simulink library "PB_Library_Master"  (R2020b)
settings: Solver=VariableStepAuto  StartTime=0.0  StopTime=10.0  RelTol=1e-3
undefined symbols (not defined in the file): A_M, B_M, E0_M, f_sw, K_M, Q_M, Q_rr, r_c, r_D, R_M, SOC_Init_M, u_ce0, u_D0
libraries: $bdroot x7, Lib_PF_BusLoadDC_TMATS x3, Lib_Dyn_StateSpace_EMTAT x3, TemperatureBlock x1
(part 1 of 3)
settings Model: Creator=nbutler2  LastModifiedBy=nbutler2

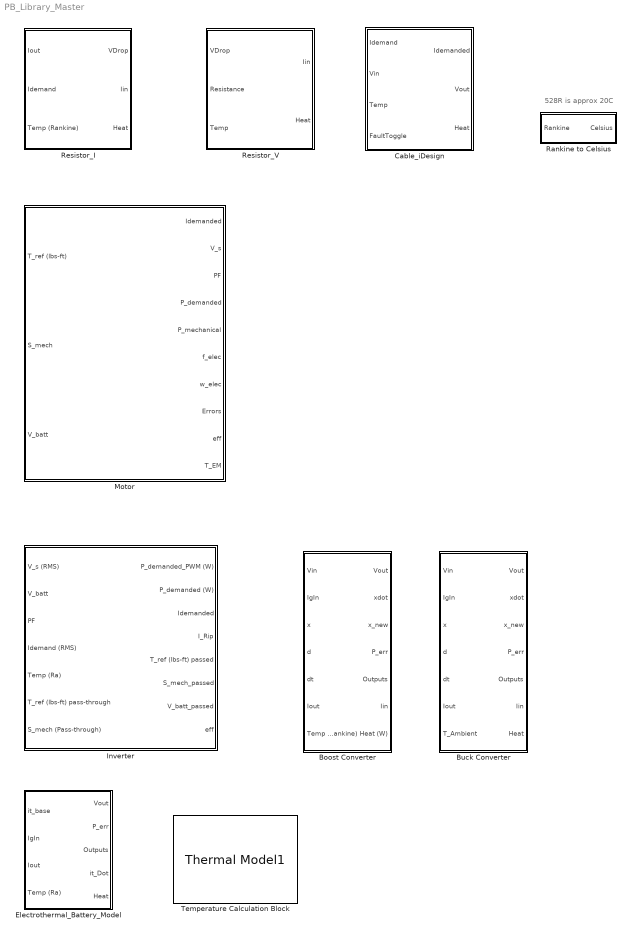
== system PB_Library_Master ==
  note: 528R is approx 20C
  Boost Converter : Subsystem  mask(DC-DC Converter){Pdis_M=1, C_M=7.5e-08, L_M=0.00058366, Ron_M=0.036, RC_M=0.13302, RL_M=0.18419, QgTotal_M=8.4e-08, Vdiode_M=1.2, TRise_M=1.72e-07, TFall_M=7.8e-08, Fsw_M=250000, Vgate_M=4, n_MOSFET=1, MassEst_M=37.515, TempIn=Celsius, vOut=1500, pow=10000, minV=490, maxV=530, rippleMode=Use defaults (5% of voltage output and 10% of inductor current), vRip=.05, iRip=.1, freqMode=Use default frequency (250 kHz), freq=250e3}
      mask prompts: Pdis_M "Pdis_M - Constant Power Leaked/Dissipated, W"; C_M "C_M - Capacitor, Farads"; L_M "L_M - Inductance, Henries"; Ron_M "Ron_M - On resistance, Ohms"; RC_M "RC_M - Resistance of Capacitor, Ohms"; RL_M "RL_M - Resistance of Inductor, Ohms"; QgTotal_M "QgTotal_M - Total Gate Charge, Coulombs"; Vdiode_M "Vdiode_M - Forward direction voltage of low-side MOSFET body diode, Volts"; TRise_M "TRise_M - Rise Time, seconds"; TFall_M "TFall_M -  Fall Time, seconds"; Fsw_M "Fsw_M - Switching frequency, Hz"; Vgate_M "Vgate_M - Gate Voltage, Volts"; n_MOSFET "Number of MOSFETs required"; MassEst_M "Mass Estimate (kg)"; TempIn "Input Units"; vOut "Desired Voltage Output"; pow "Approx. load power demand (W)"; minV "Approx. minimum input voltage"; maxV "Approx maximum input voltage"; vRip "Allowable voltage ripple as % of voltage output"; iRip "Allowable inductor current ripple as % of current output"; freq "Frequency (Hz)"
      mask help: This block represents a generic DC-DC buck converter controlled to produce a constant output voltage.The converter's efficiency is defined via a lookup table that is a function of input voltage and current. The input current is solved for, such that the power in equals the power out.
      mask init:
      | %Get current block name
      | block = gcb;
      | 
      | %Block under the mask(T_in inport)
      | block2 = [block '/T_Ambient'];
      | 
      | %Set T_in unit parameter to correct unit.
      | %switch TempIn
      | %    case 1 
      | %        set_param(block2,'Unit','degF');
      | %    case 2
      | %        set_param(block2,'Unit','degC');
      | %    case 3
      | %        set_param(block2,'Unit','degR');
      | %    case 4
      | %        set_param(block2,'Unit','K');
      | %end
      mask TypeOptions TempIn: Fahrenheit | Celsius | Rankine | Kelvin
      mask TypeOptions rippleMode: Use defaults (5% of voltage output and 10% of inductor current) | Custom value (as a nonzero % of vout and Iin)
      mask Callback rippleMode:
      | %Create mask parameter objects:
      | ripMode = get_param(gcb,'rippleMode');
      | vRip = get_param(gcb,'vRip');
      | iRip = get_param(gcb,'iRip');
      | 
      | %Returns cell array of visibility 'on'/'off' strings for all mask
      | %parameters:
      | vis = get_param(gcb,'MaskVisibilities');
      | 
      | 
      | if strcmp(ripMode(1),'C')
      |     %User selects custom ripple option:
      |     visOn = vis;
      |     %19 and 20 are the mask parameters corresponding to iRip and vRip:
      |     visOn(20:21) = {'on'};
      |     %Update mask visibilities:
      |     set_param(gcb,'MaskVisibilities',visOn);
      | else
      |     %User selects default ripple option:
      |     visOff = vis;
      |     visOff(20:21) = {'off'};
      |     set_param(gcb,'MaskVisibilities',visOff);
      |     %Set vRip and iRip to defaults:
      |     set_param(gcb,'vRip','.05');
      |     set_param(gcb,'iRip','.1');
      | end
      mask TypeOptions freqMode: Use default frequency (250 kHz) | Specify frequency
      mask Callback freqMode:
      | freqMode = get_param(gcb,'freqMode');
      | freq = get_param(gcb,'freq');
      | 
      | vis = get_param(gcb,'MaskVisibilities');
      | visOn = vis;
      | visOff = vis;
      | visOn(23) = {'on'};
      | visOff(23) = {'off'};
      | if strcmp(freqMode(1),'S')
      |     set_param(gcb,'MaskVisibilities',visOn) ;
      | else
      |     set_param(gcb,'MaskVisibilities',visOff);
      |     set_param(gcb,'freq','250e3');
      | end
      mask DialogControl Container4 Prompt: Physical Parameters
      mask DialogControl Container5 Prompt: Temperature Units
      mask DialogControl Container6 Prompt: iDesign
      mask DialogControl Container9 Prompt: New Design
      mask DialogControl runButton Prompt: RUN iDESIGN
      mask DialogControl runButton Callback:
      | %Get block handle:
      | blockHandle = getSimulinkBlockHandle(gcb);
      | 
      | 
      | %Get values of parameters and convert from string type to numeric data type:
      | V_out = str2num(get_param(blockHandle,'vOut'));
      | loadPower = str2num(get_param(blockHandle,'pow'));
      | minV_in = str2num(get_param(blockHandle,'minV'));
      | maxV_in = str2num(get_param(blockHandle,'maxV'));
      | vRippleMax = str2num(get_param(blockHandle,'vRip'));
      | iRippleMax = str2num(get_param(blockHandle,'iRip'));
      | swFreq = str2num(get_param(blockHandle,'freq'));
      | 
      | %Call iDesign_BoostConverter.m to calculate component values
      | %based on specified operating conditions:
      | [Pdis,MassEst,C,L,Ron,RC,RL,QgTotal,...
      |     VDiode, TRise,TFall,swFreq,Vgate,n_MOSFET] = ...
      |     iDesign_BoostConverter(V_out,loadPower,...
      |     minV_in,maxV_in,vRippleMax,iRippleMax,swFreq);
      | 
      | %Convert numeric data types to strings so set_param can assign them to the
      | %simulation:
      | Pdis = num2str(Pdis);
      | MassEst = num2str(MassEst);
      | C = num2str(C);
      | L = num2str(L);
      | Ron = num2str(Ron);
      | RC = num2str(RC);
      | RL = num2str(RL);
      | QgTotal = num2str(QgTotal);
      | VDiode = num2str(VDiode);
      | TRise = num2str(TRise);
      | TFall = num2str(TFall);
      | swFreq = num2str(swFreq);
      | Vgate = num2str(Vgate);
      | n_MOSFET = num2str(n_MOSFET);
      | 
      | %Set block parameters according to the values returned above:
      | set_param(blockHandle,'Pdis_M',Pdis);
      | set_param(blockHandle,'MassEst_M',MassEst);
      | set_param(blockHandle,'C_M',C);
      | set_param(blockHandle,'L_M',L);
      | set_param(blockHandle,'Ron_M',Ron);
      | set_param(blockHandle,'RC_M',RC);
      | set_param(blockHandle,'RL_M',RL);
      | set_param(blockHandle,'QgTotal_M',QgTotal);
      | set_param(blockHandle,'VDiode_M',VDiode);
      | set_param(blockHandle,'TRise_M',TRise);
      | set_param(blockHandle,'TFall_M',TFall);
      | set_param(blockHandle,'Fsw_M',swFreq);
      | set_param(blockHandle,'Vgate_M',Vgate);
      | set_param(blockHandle,'n_MOSFET',n_MOSFET);
      mask Display:
      | %switch TempIn
      | %    case 1
      | %        port_label('input', 7, 'T_Ambient (F)');
      | %    case 2
      | %        port_label('input', 7, 'T_Ambient (C)');
      | %    case 3
      | %        port_label('input', 7, 'T_Ambient (Ra)');
      | %    case 4
      | %        port_label('input', 7, 'T_Ambient (K)');
      | %end
      | 
      | port_label('input', 1, 'Vin');
      | port_label('input', 2, 'IgIn');
      | port_label('input', 3, 'x');
      | port_label('input', 4, 'd');
      | port_label('input', 5, 'dt');
      | port_label('input', 6, 'Idemand');
      | port_label('input', 7, 'Temp (Ra)');
      | 
      | 
      | port_label('output', 1, 'Vout');
      | port_label('output', 2, 'xdot');
      | port_label('output', 3, 'x_new');
      | port_label('output', 4, 'P_err');
      | port_label('output', 5, 'Outputs');
      | port_label('output', 6, 'Idemanded');
      | port_label('output', 7, 'Heat (W)');
  Buck Converter : Subsystem  mask(DC-DC Converter){Pdis_M=1, C_M=0.37515, L_M=4.4e-08, Ron_M=0.0006, RC_M=0.13, RL_M=0.286, QgTotal_M=0.18923, Vgate_M=250000, TRise_M=5e-09, TFall_M=2.3e-08, Fsw_M=2.2e-08, Trr_M=4, n_MOSFET=2.22e-07, TempIn=Celsius, vOut=50, pow=100, minV=123, maxV=127, rippleMode=Use defaults (5% of voltage output and 10% of inductor current), vRip=.05, iRip=.1, freqMode=Use default frequency (250 kHz), freq=250e3}
      mask prompts: Pdis_M "Pdis_M - Constant Power Leaked/Dissipated, W"; C_M "C_M - Capacitor, Farads"; L_M "L_M - Inductance, Henries"; Ron_M "Ron_M - On resistance, Ohms"; RC_M "RC_M - Resistance of Capacitor, Ohms"; RL_M "RL_M - Resistance of Inductor, Ohms"; QgTotal_M "QgTotal_M - Total Gate Charge, Coulombs"; Vgate_M "Vgate_M - Gate Voltage, Volts"; TRise_M "TRise_M - Rise Time, seconds"; TFall_M "TFall_M -  Fall Time, seconds"; Fsw_M "Fsw_M - Switching frequency, Hz"; Trr_M "Trr_M - Body diode reverse recovery time, seconds"; n_MOSFET "Number of MOSFETs required"; TempIn "Input Temp Units"; vOut "Desired voltage output"; pow "Approx. load power demand"; minV "Approx. minimum input voltage"; maxV "Approx. maximum input voltage"; vRip "Allowable voltage ripple as % of voltage output"; iRip "Allowable inductor current ripple as % of current output"; freq "Frequency (Hz)"
      mask help: This block represents a generic DC-DC buck converter controlled to produce a constant output voltage.The converter's efficiency is defined via a lookup table that is a function of input voltage and current. The input current is solved for, such that the power in equals the power out.
      mask init:
      | %Get current block name
      | block = gcb;
      | 
      | %Block under the mask(T_in inport)
      | block2 = [block '/T_Ambient'];
      | 
      | %Set T_in unit parameter to correct unit.
      | %switch TempIn
      | %    case 1 
      | %        set_param(block2,'Unit','degF');
      | %    case 2
      | %        set_param(block2,'Unit','degC');
      | %    case 3
      | %        set_param(block2,'Unit','degR');
      | %    case 4
      | %        set_param(block2,'Unit','K');
      | %end
      mask TypeOptions TempIn: Fahrenheit | Celsius | Rankine | Kelvin
      mask TypeOptions rippleMode: Use defaults (5% of voltage output and 10% of inductor current) | Custom value (as a nonzero % of vout and Iin)
      mask Callback rippleMode:
      | %Create mask parameter objects:
      | ripMode = get_param(gcb,'rippleMode');
      | vRip = get_param(gcb,'vRip');
      | iRip = get_param(gcb,'iRip');
      | 
      | %Returns cell array of visibility 'on'/'off' strings for all mask
      | %parameters:
      | vis = get_param(gcb,'MaskVisibilities');
      | 
      | 
      | if strcmp(ripMode(1),'C')
      |     %User selects custom ripple option:
      |     visOn = vis;
      |     %19 and 20 are the mask parameters corresponding to iRip and vRip:
      |     visOn(20:21) = {'on'};
      |     %Update mask visibilities:
      |     set_param(gcb,'MaskVisibilities',visOn);
      | else
      |     %User selects default ripple option:
      |     visOff = vis;
      |     visOff(20:21) = {'off'};
      |     set_param(gcb,'MaskVisibilities',visOff);
      |     %Set vRip and iRip to defaults:
      |     set_param(gcb,'vRip','.05');
      |     set_param(gcb,'iRip','.1');
      | end
      mask TypeOptions freqMode: Use default frequency (250 kHz) | Specify frequency
      mask Callback freqMode:
      | freqMode = get_param(gcb,'freqMode');
      | freq = get_param(gcb,'freq');
      | 
      | vis = get_param(gcb,'MaskVisibilities');
      | visOn = vis;
      | visOff = vis;
      | visOn(23) = {'on'};
      | visOff(23) = {'off'};
      | if strcmp(freqMode(1),'S')
      |     set_param(gcb,'MaskVisibilities',visOn) ;
      | else
      |     set_param(gcb,'MaskVisibilities',visOff);
      |     set_param(gcb,'freq','250e3');
      | end
      mask DialogControl Container10 Prompt: Physical Parameters
      mask DialogControl Container11 Prompt: Temperature Units
      mask DialogControl Container18 Prompt: iDesign
      mask DialogControl Container6 Prompt: New Design
      mask DialogControl Container9 Prompt: Voltage/Current Ripple
      mask DialogControl Container12 Prompt: Operating Frequency
      mask DialogControl runButton Prompt: RUN iDESIGN
      mask DialogControl runButton Callback: run iDesignMaskParamBuck.m
      mask Display:
      | %switch TempIn
      | %    case 1
      | %        port_label('input', 7, 'T_Ambient (F)');
      | %    case 2
      | %        port_label('input', 7, 'T_Ambient (C)');
      | %    case 3
      | %        port_label('input', 7, 'T_Ambient (Ra)');
      | %    case 4
      | %        port_label('input', 7, 'T_Ambient (K)');
      | %end
      | 
      | port_label('input', 1, 'Vin');
      | port_label('input', 2, 'IgIn');
      | port_label('input', 3, 'x');
      | port_label('input', 4, 'd');
      | port_label('input', 5, 'dt');
      | port_label('input', 6, 'Idemand');
      | port_label('input', 7, 'Temp (Ra)');
      | 
      | 
      | port_label('output', 1, 'Vout');
      | port_label('output', 2, 'xdot');
      | port_label('output', 3, 'x_new');
      | port_label('output', 4, 'P_err');
      | port_label('output', 5, 'Outputs');
      | port_label('output', 6, 'Idemanded');
      | port_label('output', 7, 'Heat (W)');
  Cable_iDesign : Subsystem  TreatAsAtomicUnit=on  mask{rad_c_M=0.94407, t_i_M=1.0013, Mass_M=159.0996, R_init=0.006, alpha=0.00393, V_in=120, V_drop=.3, I_out=40, Len=100, FS=1.5, Mat_c=Copper, UResis=0, UDens_C=0, UAlpha=0, Mat_i=PVC, UDens_I=0, UEpsilon=0}
      mask prompts: rad_c_M "Conductor Radius [mm]"; t_i_M "Insulator Thickness [mm]"; Mass_M "Mass [g]"; R_init "Resistance at 20C [Ohm]"; V_in "Max Voltage Input [V]"; V_drop "Allowable Voltage Drop [%]"; I_out "Max Current Output [A]"; Len "Desired Cable Length [cm]"; FS "Factor of Safety"; Mat_c "Conductor Material"; UResis "Enter Conductor Resistivity:"; UDens_C "Enter Conductor Density:"; UAlpha "Enter Conductor Thermal Coefficient:"; Mat_i "Insulator Material"; UDens_I "Enter Insulator Density:"; UEpsilon "Enter Insulator Dielectric Permittivity:"
      mask init:
      | %Get current block name
      | %block = gcb;
      | 
      | %Block under the mask(T_in inport and outport)
      | %block2 = [block '/T_in'];
      | 
      | %Set T_in unit parameter to correct unit.
      | %{
      | switch TempIn
      |     case 1 
      |         set_param(block2,'Unit','degF');
      |     case 2
      |         set_param(block2,'Unit','degC');
      |     case 3
      |         set_param(block2,'Unit','degR');
      |     case 4
      |         set_param(block2,'Unit','K');
      | end
      | %}
      mask TypeOptions Mat_c: Copper | Aluminum | Steel | User-Defined
      mask Callback Mat_c:
      | % Get the mask parameter values. This is a cell
      | %   array of character vectors.
      | maskStrC = get_param(gcb,'Mat_c');
      | maskStrI = get_param(gcb,'Mat_i');
      | 
      | % The pop-up menu is the first mask parameter.
      | %   Check the value selected in the pop-up
      | if strcmp(maskStrC(1),'U') & strcmp(maskStrI(1),'U')
      | 
      |     % Set the visibility of both parameters on when
      |     %   User-defined is selected in the pop-up.
      | 
      |     set_param(gcb,'MaskVisibilities',{'on';'on';'on';'on'; 'off'   %Physical parameters
      |         'on';'on';'on';'on';'on';   %iDesign cable general properties
      |         'on';'on';'on';'on';'on';'on';'on'})     %Material Properties
      | 
      | elseif strcmp(maskStrC(1),'U') & ~strcmp(maskStrI(1),'U')
      | 
      |     % Turn off the visibility of the Value field
      |     %   when User-defined is not selected.
      | 
      |     set_param(gcb,'MaskVisibilities',{'on';'on';'on';'on';'off';    %Physical parameters
      |         'on';'on';'on';'on';'on';   %iDesign cable general properties
      |         'on';'on';'on';'on';'on';'off';'off'})     %Material Properties
      | 
      | 
      | elseif ~strcmp(maskStrC(1),'U') & strcmp(maskStrI(1),'U')
      | 
      |     % Turn off the visibility of the Value field
      |     %   when User-defined is not selected.
      | 
      |     set_param(gcb,'MaskVisibilities',{'on';'on';'on';'on';'off';    %Physical parameters
      |         'on';'on';'on';'on';'on';   %iDesign cable general properties
      |         'on';'off';'off';'off';'on';'on';'on'})     %Material Properties
      | 
      | else
      | 
      |     % Turn off the visibility of the Value field
      |     %   when User-defined is not selected.
      | 
      |     set_param(gcb,'MaskVisibilities',{'on';'on';'on';'on';'off';    %Physical parameters
      |         'on';'on';'on';'on';'on';   %iDesign cable general properties
      |         'on';'off';'off';'off';'on';'off';'off'})     %Material Properties
      | 
      |     % Set the character vector in the Values field equal to the
      |     % character vector selected in the Gain pop-up menu.
      | 
      |     %maskStr{2}=maskStr{1};
      |     %set_param(gcb,'editValue',maskStr);
      | end
      mask TypeOptions Mat_i: PVC | PE | ETFE | User-Defined
      mask Callback Mat_i:
      | % Get the mask parameter values. This is a cell
      | %   array of character vectors.
      | maskStrC = get_param(gcb,'Mat_c');
      | maskStrI = get_param(gcb,'Mat_i');
      | 
      | % The pop-up menu is the first mask parameter.
      | %   Check the value selected in the pop-up
      | if strcmp(maskStrC(1),'U') & strcmp(maskStrI(1),'U')
      | 
      |     % Set the visibility of both parameters on when
      |     %   User-defined is selected in the pop-up.
      | 
      |     set_param(gcb,'MaskVisibilities',{'on';'on';'on';'on';'off';    %
      |         'on';'on';'on';'on';'on';   %iDesign cable general properties
      |         'on';'on';'on';'on';'on';'on';'on'})     %Material Properties
      | 
      | elseif strcmp(maskStrC(1),'U') & ~strcmp(maskStrI(1),'U')
      | 
      |     % Turn off the visibility of the Value field
      |     %   when User-defined is not selected.
      | 
      |     set_param(gcb,'MaskVisibilities',{'on';'on';'on';'on';'off';    %
      |         'on';'on';'on';'on';'on';   %iDesign cable general properties
      |         'on';'on';'on';'on';'on';'off';'off'})     %Material Properties
      | 
      | 
      | elseif ~strcmp(maskStrC(1),'U') & strcmp(maskStrI(1),'U')
      | 
      |     % Turn off the visibility of the Value field
      |     %   when User-defined is not selected.
      | 
      |     set_param(gcb,'MaskVisibilities',{'on';'on';'on';'on';'off';    %
      |         'on';'on';'on';'on';'on';   %iDesign cable general properties
      |         'on';'off';'off';'off';'on';'on';'on'})     %Material Properties
      | 
      | else
      | 
      |     % Turn off the visibility of the Value field
      |     %   when User-defined is not selected.
      | 
      |     set_param(gcb,'MaskVisibilities',{'on';'on';'on';'on';'off';    %
      |         'on';'on';'on';'on';'on';   %iDesign cable general properties
      |         'on';'off';'off';'off';'on';'off';'off'})     %Material Properties
      | 
      |     % Set the character vector in the Values field equal to the
      |     % character vector selected in the Gain pop-up menu.
      | 
      |     %maskStr{2}=maskStr{1};
      |     %set_param(gcb,'editValue',maskStr);
      | end
      mask DialogControl Container4 Prompt: Parameters
      mask DialogControl Container5 Prompt: iDesign
      mask DialogControl Container7 Prompt: New Design
      mask DialogControl runButton Prompt: RUN iDESIGN
      mask DialogControl runButton Callback:
      | %Get block handle:
      | blockHandle = getSimulinkBlockHandle(gcb);
      | 
      | %Get values of parameters and convert from string type to numeric data type:
      | V_in = str2num(get_param(blockHandle, 'V_in'));
      | V_drop = str2num(get_param(blockHandle, 'V_drop'));
      | I_out = str2num(get_param(blockHandle, 'I_out'));
      | Length = str2num(get_param(blockHandle, 'Len'));
      | Derat_Fact = str2num(get_param(blockHandle, 'FS'));
      | 
      | Mat_c = get_param(blockHandle, 'Mat_c');
      | UResis = str2num(get_param(blockHandle, 'UResis'));
      | UDens_C = str2num(get_param(blockHandle, 'UDens_C'));
      | UAlpha = str2num(get_param(blockHandle, 'UAlpha'));
      | 
      | Mat_i = get_param(blockHandle, 'Mat_i');
      | UDens_I = str2num(get_param(blockHandle, 'UDens_I'));
      | UEpsilon = str2num(get_param(blockHandle, 'UEpsilon'));
      | 
      | 
      | %Call iDesign_Cable.m to calculate component values
      | %based on specified operating conditions:
      | 
      | [radius_c, t_i, Mass, R_c, alpha] = iDesign_Cable(V_in, V_drop,...
      |     I_out, Length, Mat_c, UResis, UDens_C, UAlpha,...
      |     Mat_i, UDens_I, UEpsilon, Derat_Fact);
      | 
      | %Convert numeric data types to strings so set_param
      | %can assign them to the simulation:
      | radius_c = num2str(radius_c);
      | t_i = num2str(t_i);
      | Mass = num2str(Mass);
      | R_init = num2str(R_c);
      | alpha = num2str(alpha);
      | 
      | %Set block parameters according to the values returned above:
      | set_param(blockHandle, 'rad_c_M', radius_c);
      | set_param(blockHandle, 't_i_M', t_i);
      | set_param(blockHandle, 'Mass_M', Mass);
      | set_param(blockHandle, 'R_init', R_init);
      | set_param(blockHandle, 'alpha', alpha);
      mask Display:
      | port_label('input', 1, 'I_demand');
      | port_label('input', 2, 'Vin');
      | port_label('input', 3, 'Temp (Ra)');
      | port_label('input', 4, 'FaultToggle');
      | 
      | port_label('output', 1, 'I_demanded');
      | port_label('output', 2, 'VOut');
      | port_label('output', 3, 'Heat (W)');
  Electrothermal_Battery_Model : Subsystem  mask(HiFiBattery){E0_M=E0_M, Q_M=Q_M, R_M=R_M, K_M=K_M, B_M=B_M, SOC_Init_M=SOC_Init_M, A_M=A_M, battery_type_M=Li-Ion, batt_mass_field=0, TempIn=Celsius, BWS=on, thermal=on, nameField=Thermal Model}
      mask prompts: E0_M "E0_M – battery constant voltage (V)"; Q_M "Q_M – battery capacity (Ah)"; R_M "R_M – battery internal resistance (ohm)"; K_M "K_M – polarization constant (Ah^-1)"; B_M "B_M – exponential zone time constant inverse (Ah^-1)"; SOC_Init_M "SOC_Init_M – initial percentage state of charge (%)"; A_M "A_M – exponential zone amplitude (V)"; battery_type_M "battery_type_M - Li-Ion-, Ni-MH-, or Lead Acid-based chemistry"; batt_mass_field "Approximate battery mass (0=N/A)"; TempIn "Input Temp Units:"; BWS "Load Parameters into Base Workspace"; thermal "Load Thermal Block parameters when loading battery block parameters"; nameField "Name of thermal block coupled with battery block:"
      mask help: This block represents a physics-based battery model. The output voltage is a function of the current drawn from the battery ('Iout'), and the time integral of the current drawn from the battery, ('it', in Amp-hours). You need an integrator that takes in it_dot, and you need to feed that integrated it value into it_base. The initial condition for it_base should be zero, as this integrator should keep track of consumed charge, in amp-hours. If you put in a value other than 100% for SOC_Init_M, then you will see a difference between the it_base (which always starts at zero), and it as you get it from the Outputs structure, which accounts for the difference in SOC_Init_M from 100%.
      mask init:
      | %Get current block name
      | block = gcb;
      | 
      | %Block under the mask(T_in inport)
      | %block2 = [block '/T_avg'];
      | %Set T_in unit parameter to correct unit.
      | %switch TempIn
      | %    case 1 
      | %        set_param(block2,'Unit','degF');
      | %    case 2
      | %        set_param(block2,'Unit','degC');
      | %    case 3
      | %        set_param(block2,'Unit','degR');
      | %    case 4
      | %        set_param(block2,'Unit','K');
      | %end
      mask TypeOptions battery_type_M: Li-Ion | Ni-MH/Lead Acid
      mask TypeOptions TempIn: Fahrenheit | Celsius | Rankine | Kelvin
      mask Callback thermal:
      | thermal = get_param(gcb,'thermal');
      | %Returns cell array of visibility 'on'/'off' strings for all mask
      | %parameters:
      | vis = get_param(gcb,'MaskVisibilities');
      | 
      | 
      | if strcmp(thermal,'on')
      |     visOn = vis;
      |     visOn(13) = {'on'};
      |     set_param(gcb,'MaskVisibilities',visOn);
      | else
      |     visOff = vis;
      |     visOff(13) = {'off'};
      |     set_param(gcb,'MaskVisibilities',visOff);
      | end
      mask DialogControl TempGroupVar Prompt: Temperature Units
      mask DialogControl Container7 Prompt: iDesign
      mask DialogControl Control2 Prompt: Open Design GUI
      mask DialogControl Control2 Callback: run('Battery_Discharge_exported');
      mask DialogControl Control3 Prompt: Load Parameters
      mask DialogControl Control3 Callback:
      | file = uigetfile('.mat');
      | BWS = get_param(gcb,'BWS');
      | %Set Thermal block's parameters if selected
      | thermal = get_param(gcb,'thermal');
      | modelPath = gcs;
      | nameField = get_param(gcb,'nameField');
      | thermalPath = strcat(modelPath,'/',nameField);
      | 
      | if strcmp(BWS,'on')
      |     %Load variables into base workspace and use them as block parameters:
      |     batt = open(file);
      | 
      |     assignin('base','Q_M',batt.Q_M);
      |     assignin('base','A_M',batt.A_M);
      |     assignin('base','B_M',batt.B_M);
      |     assignin('base','R_M',batt.R_M);
      |     assignin('base','K_M',batt.K_M);
      |     assignin('base','E0_M',batt.E0_M);
      |     assignin('base','SOC_Init_M',batt.SOC_Init_M);
      | %     if exist(batt_mass) = 1
      | %         assignin('base','batt_mass',batt.batt_mass);
      | %     else
      | %         assignin('base',batt_mass',0);
      | %     end
      |     %Set battery block's parameters:
      |     assignin('base','batt_mass',batt.batt_mass);
      |     set_param(gcb,'E0_M','E0_M');
      |     set_param(gcb,'Q_M','Q_M');
      |     set_param(gcb,'R_M','R_M');
      |     set_param(gcb,'K_M','K_M');
      |     set_param(gcb,'B_M','B_M');
      |     set_param(gcb,'A_M','A_M');
      |     set_param(gcb,'SOC_Init_M','SOC_Init_M');
      | 
      | 
      | 
      |     if strcmp(thermal,'on')
      |         %Thermal block parameters:
      |         assignin('base','Cj_M',batt.Cj_M);
      |         assignin('base','Cs_M',batt.Cs_M);
      |         assignin('base','Ts_0_M',batt.Ts_0_M);
      |         assignin('base','Tj_0_M',batt.Tj_0_M);
      |         assignin('base','Ru_M',batt.Ru_M);
      |         assignin('base','Rj_M',batt.Rj_M);
      | 
      |         set_param(thermalPath,'Cs_M','Cs_M');
      |         set_param(thermalPath,'Ru_M','Ru_M');
      |         set_param(thermalPath,'Ts_0_M','Ts_0_M');
      |         set_param(thermalPath,'Cj_M','Cj_M');
      |         set_param(thermalPath,'Rj_M','Rj_M');
      |         set_param(thermalPath,'Tj_0_M','Tj_0_M');
      |     end
      | else
      |     %Use the values from the parameter file as the block parameters without
      |     %saving them in the base workspace (no worries about overwriting other
      |     %existing variables):
      |     batt = open(file);
      |     Q = num2str(batt.Q_M);
      |     A = num2str(batt.A_M);
      |     B = num2str(batt.B_M);
      |     R = num2str(batt.R_M);
      |     K = num2str(batt.K_M);
      |     E0 = num2str(batt.E0_M);
      |     SOC_Init = num2str(batt.SOC_Init_M);
      |     Cs = num2str(batt.Cs_M);
      |     Ru = num2str(batt.Ru_M);
      |     Ts = num2str(batt.Ts_0_M);
      |     Cj = num2str(batt.Cj_M);
      |     Rj = num2str(batt.Rj_M);
      |     Tj = num2str(batt.Tj_0_M);
      |     batt_mass = num2str(batt.batt_mass);
      | 
      |     set_param(gcb,'E0_M',E0);
      |     set_param(gcb,'Q_M',Q);
      |     set_param(gcb,'R_M',R);
      |     set_param(gcb,'K_M',K);
      |     set_param(gcb,'B_M',B);
      |     set_param(gcb,'A_M',A);
      |     set_param(gcb,'SOC_Init_M',SOC_Init);
      |     set_param(gcb,'batt_mass_field',batt_mass);
      |     if strcmp(thermal,'on')
      |         set_param(thermalPath,'Cs_M',Cs);
      |         set_param(thermalPath,'Ru_M',Ru);
      |         set_param(thermalPath,'Ts_0_M',Ts);
      |         set_param(thermalPath,'Cj_M',Cj);
      |         set_param(thermalPath,'Rj_M',Rj);
      |         set_param(thermalPath,'Tj_0_M',Tj);
      |     end
      | 
      | 
      | end
      mask Display:
      | port_label('input', 1, 'it_base');
      | port_label('input', 2, 'Igin');
      | port_label('input', 3, 'Iout');
      | port_label('input', 4, 'Temp (Ra)');
      | 
      | port_label('output', 1, 'Vout');
      | port_label('output', 2, 'P_err');
      | port_label('output', 3, 'Outputs');
      | port_label('output', 4, 'it_Dot');
      | port_label('output', 5, 'Heat (W)');
  Inverter : Subsystem  mask{T_M=[25 175], u_D_M=[1.16666666666667 0.999999999999998], u_ce0_M=[0.971428571428571 0.848275862068965], R_c_M=[0.0285714285714286 0.0551724137931034], R_D_M=[0.0238095238095238 0.0294117647058824], E0_M=[6.00000000000002e-05 6.00000000000002e-05], E1_M=[5.6e-05 5.6e-05], f_sw_M=20000, L_s_M=0.1, P_max_I=22000, V_phase_I=600, f_sw_I=0, L_s_I=0.1}
      mask prompts: T_M "Temperature Breakpoints (degrees C)"; u_D_M "u_D (Diode voltage at 0A), as a function of T"; u_ce0_M "u_ce0 (IGBT voltage at 0A), as a function of T"; R_c_M "R_c (IGBT resistance), as a function of T"; R_D_M "R_D (Diode resistance), as a linear of T"; E0_M "E0 switching energy coefficient"; E1_M "E1 switching energy coefficient"; f_sw_M "Switching Frequency (Hz)"; L_s_M "Stator Inductance of Attached Motor"; P_max_I "Maximum power"; V_phase_I "Maximum phase voltage (set to 0 to disregard)"; f_sw_I "F_sw (set to 0 to default to maximum for given IGBT)"; L_s_I "Stator inductance of Motor (required for ripple current calculation)"
      mask DialogControl Container4 Prompt: Parameters
      mask DialogControl Control2 Prompt: The way that the above parameters are used is that each vector is 2 long, using points in the linear zone of the curves. Interpolation is used to find values at other temperatures.
      mask DialogControl Container4_copy Prompt: iDesign 1
      mask DialogControl runbutton Prompt: RUN iDESIGN
      mask DialogControl runbutton Callback: run('Run_iDesign_InverterSS')
  Motor : Subsystem  mask{pp=2.5, flux_m=0.46219, R_s=0.032, L_s=0.00115, P_Fe_Nom=-16822495.6386, S_nom=3000, T_nom=94.906, P_out_max=16845400, I_max=36.5, P_in_max=30000, T_max=108.464, MassEst_M=-1080970, Poles_i=5, R_s_i=.032, L_s_i=.00086+0.00029, S_nom_i=3000, T_nom_i=70, P_out_max_i=22000, I_max_i=36.5, P_in_max_i=30000, K_i=121, V_nom_i=368, T_max_i=80, CalculatePFe=Compute iron losses automatically, P_Fe_Nom_i=0, I_nom_i=36.5, PF_nom_i=0.99, P_Fe_Calc_Flag=1}
      mask prompts: pp "Pole Pairs"; flux_m "Magnet Flux (wb)"; R_s "Stator Resistance (Ohm)"; L_s "Stator Inductance (H)"; P_Fe_Nom "Iron Losses at Nominal Speed (W)"; S_nom "Nominal Speed (RPM)"; T_nom "Maximum/Nominal reference torque (lbs-ft)"; P_out_max "Maximum output power (W)"; I_max "Currrent Limit"; P_in_max "Input power limit"; T_max "Maximum allowable torque"; MassEst_M "Weight Estimate (kg)"; Poles_i "Number of poles"; R_s_i "Stator Resistance (Ohm)"; L_s_i "Stator Inductance (H)"; S_nom_i "Nominal Speed (RPM)"; T_nom_i "Maximum/Nominal reference torque (lbs-ft)"; P_out_max_i "Maximum output power (W)"; I_max_i "Currrent Limit"; P_in_max_i "Input power limit"; K_i "Back EMF Constant (V/kRPM)"; V_nom_i "Nominal Voltage"; T_max_i "Maximum allowable torque"; P_Fe_Nom_i "Iron Loss at Nominal Conditions"; I_nom_i "Nominal Current"; PF_nom_i "Nominal power factor"
      mask TypeOptions CalculatePFe: Compute iron losses automatically | Input iron losses manually
      mask Callback CalculatePFe:
      | %Create mask parameter objects:
      | PFeMode = get_param(gcb,'CalculatePFe');
      | % P_Fe_Calc_Flag = get_param(gcb,'P_Fe_Calc_Flag');
      | 
      | %Returns cell array of visibility 'on'/'off' strings for all mask
      | %parameters:
      | vis = get_param(gcb,'MaskVisibilities');
      | 
      | if strcmp(PFeMode(1),'I') == 1
      |     %User selects custom ripple option:
      |     visOn = vis;
      |     visOn(24) = {'on'};
      |     visOn(25) = {'off'};
      |     visOn(26) = {'off'};
      |     visOn(27) = {'off'};
      |     %Update mask visibilities:
      |     set_param(gcb,'MaskVisibilities',visOn);
      |     Calculate_Pe_Fe_Flag = 0;
      |     set_param(gcb,'P_Fe_Calc_Flag','0');
      | else
      |     visOff = vis;
      |     visOff(24) = {'off'};
      |     visOff(25) = {'on'};
      |     visOff(26) = {'on'};
      |     visOff(27) = {'off'};
      |     Calculate_Pe_Fe_Flag = 1;
      |     set_param(gcb,'MaskVisibilities',visOff);
      |     set_param(gcb,'P_Fe_Calc_Flag','1');
      | end
      mask DialogControl Container13 Prompt: Parameters
      mask DialogControl Container12 Prompt: iDesign
      mask DialogControl Control3 Prompt: Entering zero for resistance or inductance will cause iDesign to use statistical analysis of a set of 400V PMSMs in order to estimate a reasonable resistance and inductance.
      mask DialogControl Container14 Prompt: Iron Loss Calculation
      mask DialogControl run Prompt: RUN IDESIGN
      mask DialogControl run Callback: run('Run_iDesign_SS_PMSM_USUnits')
  Rankine to Celsius : Subsystem
  Resistor_I : Subsystem  mask{TempIn=Celsius}
      mask prompts: TempIn "Input Units"
      mask init:
      | %Get current block name
      | block = gcb;
      | 
      | %Block under the mask(T_in inport and outport)
      | %block2 = [block '/T_in'];
      | 
      | %Set T_in unit parameter to correct unit.
      | %switch TempIn
      | %    case 1 
      | %        set_param(block2,'Unit','degF');
      | %    case 2
      | %        set_param(block2,'Unit','degC');
      | %    case 3
      | %        set_param(block2,'Unit','degR');
      | %    case 4
      | %        set_param(block2,'Unit','K');
      | %end
      mask TypeOptions TempIn: Fahrenheit | Celsius | Rankine | Kelvin
      mask DialogControl Container4 Prompt: Parameters
      mask DialogControl Container8 Prompt: Temperature Units
      mask Display:
      | port_label('input', 1, 'Idemand');
      | port_label('input', 2, 'Resistance');
      | port_label('input', 3, 'Temp (Ra)');
      | 
      | port_label('output', 1, 'VDrop');
      | port_label('output', 2, 'Idemanded');
      | port_label('output', 3, 'Heat (W)');
  Resistor_V : Subsystem  mask{TempIn=Celsius}
      mask prompts: TempIn "Input Units"
      mask init:
      | %Get current block name
      | block = gcb;
      | 
      | %Block under the mask(T_in inport and outport)
      | block2 = [block '/T_in'];
      | 
      | %Set T_in unit parameter to correct unit.
      | %switch TempIn
      | %    case 1 
      | %        set_param(block2,'Unit','degF');
      | %    case 2
      | %        set_param(block2,'Unit','degC');
      | %    case 3
      | %        set_param(block2,'Unit','degR');
      | %    case 4
      | %        set_param(block2,'Unit','K');
      | %end
      mask TypeOptions TempIn: Fahrenheit | Celsius | Rankine | Kelvin
      mask DialogControl Container4 Prompt: Parameters
      mask DialogControl Container6 Prompt: Temperature Units
      mask Display:
      | port_label('input', 1, 'VDrop');
      | port_label('input', 2, 'Resistance');
      | port_label('input', 3, 'Temp (Ra)');
      | 
      | 
      | port_label('output', 1, 'Idemand');
      | port_label('output', 2, 'Heat (W)');
  Temperature Calculation Block : TemperatureBlock/Thermal Model1  Tj_0_M=25  Ts_0_M=25  Cj_M=Cj  Rj_M=Rj  Ru_M=Ru  Cs_M=Cs

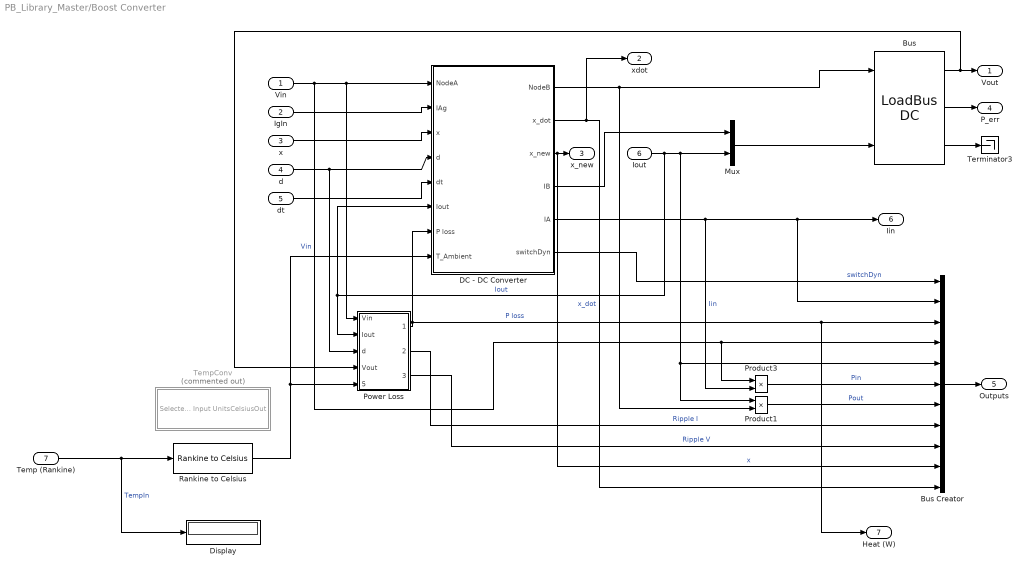
== system PB_Library_Master/Boost Converter ==
  Vin : Inport
  IgIn : Inport  Port=2
  x : Inport  Port=3
  d : Inport  Port=4
  dt : Inport  Port=5
  Iout : Inport  Port=6
  Temp (Rankine) : Inport  Port=7  Unit=degC
  Bus : Lib_PF_BusLoadDC_TMATS/LoadBus DC  P_M=-Pdis_M  BlkNm_M=double(gcb)
  Bus Creator : BusCreator  Inputs=11
  DC - DC Converter : Subsystem
      mask Display:
      | fprintf('Boost')
      | 
      | port_label('input',1,'VA')
      | port_label('input',2,'IAg')
      | port_label('input',3,'x')
      | port_label('input',4,'d')
      | port_label('input',5,'dt')
      | port_label('input',6,'Iout')
      | port_label('input',7,'Ploss')
      | 
      | 
      | port_label('output',1,'VB')
      | port_label('output',2,'x_dot')
      | port_label('output',3,'x_new')
      | port_label('output',4,'IB')
      | port_label('output',5,'IA')
      | port_label('output',6,'switchDyn')
  Display : Display
  Mux : Mux  Inputs=2
  "Power Loss " : Subsystem
  Product1 : Product
  Product3 : Product
  Rankine to Celsius : $bdroot/Rankine to Celsius  SystemSampleTime=-1  VariantActivationTime=update diagram  Latency=0  AutoFrameSizeCalculation=off
  "TempConv " : Subsystem  Commented=on
      mask DialogControl DescTextVar Prompt: Temperature Unit Converter
  Terminator3 : Terminator
  Vout : Outport  VectorParamsAs1DForOutWhenUnconnected=off
  xdot : Outport  Port=2  VectorParamsAs1DForOutWhenUnconnected=off
  x_new : Outport  Port=3  VectorParamsAs1DForOutWhenUnconnected=off
  P_err : Outport  Port=4  VectorParamsAs1DForOutWhenUnconnected=off
  Outputs : Outport  Port=5  VectorParamsAs1DForOutWhenUnconnected=off
  Iin : Outport  Port=6  VectorParamsAs1DForOutWhenUnconnected=off
  Heat (W) : Outport  Port=7  VectorParamsAs1DForOutWhenUnconnected=off
  wires:
  Temp (Rankine)/1 -> Rankine to Celsius/1, Display/1  "TempIn"
  Rankine to Celsius/1 -> DC - DC Converter/8("T_Ambient "), "Power Loss "/5("T_Ambient ")
  DC - DC Converter/6(switchDyn) -> Bus Creator/1  "switchDyn"
  dt/1 -> DC - DC Converter/5(dt)
  DC - DC Converter/3(x_new) -> x_new/1, Bus Creator/10  "x"
  "Power Loss "/1(" P loss") -> Heat (W)/1, Bus Creator/3, DC - DC Converter/7(P loss)  "P loss"
  d/1 -> "Power Loss "/3(d), DC - DC Converter/4(d)
  x/1 -> DC - DC Converter/3(x)
  IgIn/1 -> DC - DC Converter/2(IAg)
  DC - DC Converter/5(IA) -> Iin/1, Bus Creator/2, Product3/2  "Iin"
  DC - DC Converter/4(IB) -> Mux/1
  DC - DC Converter/2(x_dot) -> xdot/1, Bus Creator/11  "x_dot"
  Iout/1 -> Mux/2, Bus Creator/5, Product1/1, "Power Loss "/2(Iout), DC - DC Converter/6(Iout)  "Iout"
  Bus/1 -> Vout/1, "Power Loss "/4(Vout)
  Product1/1 -> Bus Creator/7  "Pout"
  Product3/1 -> Bus Creator/6  "Pin"
  Vin/1 -> Bus Creator/4, Product3/1, "Power Loss "/1(Vin), DC - DC Converter/1(NodeA)  "Vin"
  DC - DC Converter/1(NodeB) -> Bus/1, Product1/2
  Bus/3 -> Terminator3/1
  Bus/2 -> P_err/1
  Bus Creator/1 -> Outputs/1
  "Power Loss "/3(RippleV) -> Bus Creator/9  "Ripple V"
  "Power Loss "/2(RippleI) -> Bus Creator/8  "Ripple I"
  Mux/1 -> Bus/3

== system PB_Library_Master/Buck Converter ==
  Vin : Inport
  IgIn : Inport  Port=2
  x : Inport  Port=3
  d : Inport  Port=4
  dt : Inport  Port=5
  Iout : Inport  Port=6
  T_Ambient : Inport  Port=7  Unit=degC
  Bus : Lib_PF_BusLoadDC_TMATS/LoadBus DC  P_M=-Pdis_M  BlkNm_M=double(gcb)
  Bus Creator : BusCreator  Inputs=11
  DC - DC Converter : Subsystem
      mask Display:
      | fprintf('Buck')
      | 
      | port_label('input',1,'VA')
      | port_label('input',2,'IAg')
      | port_label('input',3,'x')
      | port_label('input',4,'d')
      | port_label('input',5,'dt')
      | port_label('input',6,'Iout')
      | port_label('input',7,'Ploss')
      | 
      | 
      | port_label('output',1,'VB')
      | port_label('output',2,'x_dot')
      | port_label('output',3,'x_new')
      | port_label('output',4,'IB')
      | port_label('output',5,'IA')
      | port_label('output',6,'switchDyn')
  Mux : Mux  Inputs=2
  "Power Loss " : Subsystem
  Product1 : Product
  Product3 : Product
  Rankine to Celsius : $bdroot/Rankine to Celsius  SystemSampleTime=-1  VariantActivationTime=update diagram  Latency=0  AutoFrameSizeCalculation=off
  "TempConv " : Subsystem  Commented=on
      mask DialogControl DescTextVar Prompt: Temperature Unit Converter
  Terminator3 : Terminator
  Vout : Outport  VectorParamsAs1DForOutWhenUnconnected=off
  xdot : Outport  Port=2  VectorParamsAs1DForOutWhenUnconnected=off
  x_new : Outport  Port=3  VectorParamsAs1DForOutWhenUnconnected=off
  P_err : Outport  Port=4  VectorParamsAs1DForOutWhenUnconnected=off
  Outputs : Outport  Port=5  VectorParamsAs1DForOutWhenUnconnected=off
  Iin : Outport  Port=6  VectorParamsAs1DForOutWhenUnconnected=off
  Heat : Outport  Port=7  VectorParamsAs1DForOutWhenUnconnected=off
  wires:
  Rankine to Celsius/1 -> DC - DC Converter/8("T_Ambient "), "Power Loss "/5("T_Ambient ")
  T_Ambient/1 -> Rankine to Celsius/1
  DC - DC Converter/6(switchDyn) -> Bus Creator/1  "switchDyn"
  dt/1 -> DC - DC Converter/5(dt)
  DC - DC Converter/3(x_new) -> x_new/1, Bus Creator/10  "x"
  "Power Loss "/1(" P loss") -> Bus Creator/3, Heat/1, DC - DC Converter/7(P loss)  "P loss"
  d/1 -> "Power Loss "/3(d), DC - DC Converter/4(d)
  x/1 -> DC - DC Converter/3(x)
  DC - DC Converter/5(IA) -> Iin/1, Bus Creator/2, Product3/2  "Iin"
  DC - DC Converter/4(IB) -> Mux/1
  DC - DC Converter/2(x_dot) -> xdot/1, Bus Creator/11  "x_dot"
  Iout/1 -> Mux/2, Bus Creator/5, Product1/1, "Power Loss "/2(Iout), DC - DC Converter/6(Iout)  "Iout"
  Bus/1 -> "Power Loss "/4(Vout), Vout/1
  Product1/1 -> Bus Creator/7  "Pout"
  Product3/1 -> Bus Creator/6  "Pin"
  DC - DC Converter/1(NodeB) -> Bus/1, Product1/2
  Bus/3 -> Terminator3/1
  Bus/2 -> P_err/1
  Bus Creator/1 -> Outputs/1
  "Power Loss "/3(RippleV) -> Bus Creator/9  "Ripple V"
  "Power Loss "/2(RippleI) -> Bus Creator/8  "Ripple I"
  Mux/1 -> Bus/3
  IgIn/1 -> DC - DC Converter/2(IAg)
  Vin/1 -> Bus Creator/4, Product3/1, "Power Loss "/1(Vin), DC - DC Converter/1(NodeA)  "Vin"

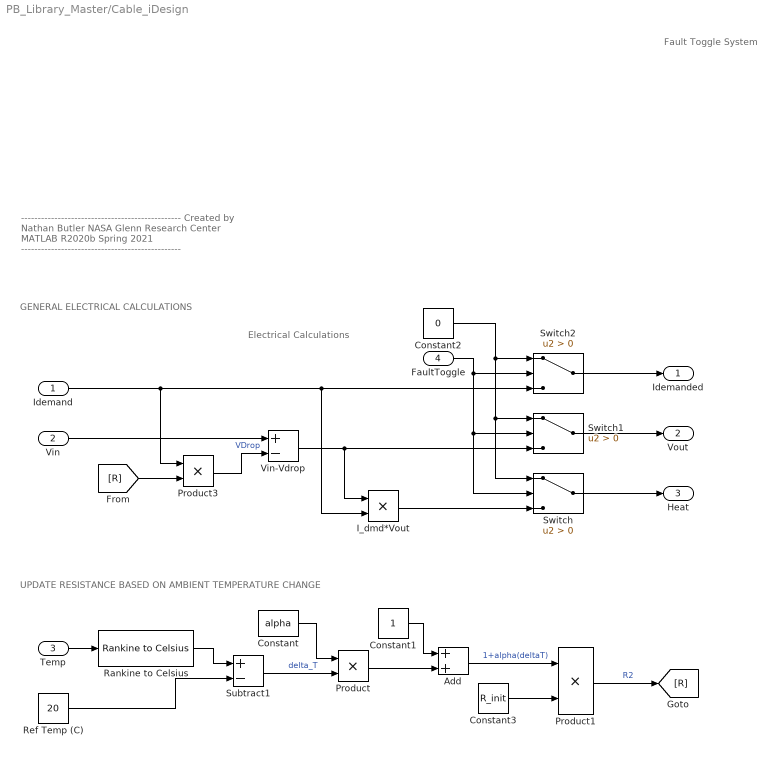
== system PB_Library_Master/Cable_iDesign ==
  note: Electrical Calculations
  note: Fault Toggle System
  note: UPDATE RESISTANCE BASED ON AMBIENT TEMPERATURE CHANGE
  note: GENERAL ELECTRICAL CALCULATIONS
  note: ------------------------------------------------
      | Created by Nathan Butler
      | NASA Glenn Research Center
      | MATLAB R2020b
      | Spring 2021
      | ------------------------------------------------
  Idemand : Inport
  Vin : Inport  Port=2
  Temp : Inport  Port=3
  FaultToggle : Inport  Port=4
  Add : Sum
  Constant : Constant  Value=alpha
  Constant1 : Constant
  Constant2 : Constant  Value=0
  Constant3 : Constant  Value=R_init
  I_dmd*Vout : Product
  Product : Product
  Product1 : Product
  Product3 : Product
  Rankine to Celsius : $bdroot/Rankine to Celsius  SystemSampleTime=-1  VariantActivationTime=update diagram  Latency=0  AutoFrameSizeCalculation=off
  Ref Temp (C) : Constant  Value=20
  Subtract1 : Sum  Inputs=+-
  Switch : Switch  Criteria=u2 > Threshold
  Switch1 : Switch  Criteria=u2 > Threshold
  Switch2 : Switch  Criteria=u2 > Threshold
  Vin-Vdrop : Sum  Inputs=+-
  Idemanded : Outport  VectorParamsAs1DForOutWhenUnconnected=off
  Vout : Outport  Port=2  VectorParamsAs1DForOutWhenUnconnected=off
  Heat : Outport  Port=3  VectorParamsAs1DForOutWhenUnconnected=off
  wires:
  Vin/1 -> Vin-Vdrop/1
  Subtract1/1 -> Product/2  "delta_T"
  Constant/1 -> Product/1
  Product/1 -> Add/2
  Constant1/1 -> Add/1
  Add/1 -> Product1/1  "1+alpha(deltaT)"
  Product1/1 -> [R]  "R2"
  Constant3/1 -> Product1/2
  Ref Temp (C)/1 -> Subtract1/2
  Vin-Vdrop/1 -> I_dmd*Vout/1, Switch1/3
  Idemand/1 -> Product3/1, I_dmd*Vout/2, Switch2/3
  [R] -> Product3/2
  Product3/1 -> Vin-Vdrop/2  "VDrop"
  Switch1/1 -> Vout/1
  Switch2/1 -> Idemanded/1
  I_dmd*Vout/1 -> Switch/3
  Switch/1 -> Heat/1
  Constant2/1 -> Switch2/1, Switch/1, Switch1/1
  FaultToggle/1 -> Switch1/2, Switch/2, Switch2/2
  Temp/1 -> Rankine to Celsius/1
  Rankine to Celsius/1 -> Subtract1/1

== system PB_Library_Master/Electrothermal_Battery_Model ==
  note: Electrical Model
  note: Bus Library Block
  it_base : Inport
  IgIn : Inport  Port=2
  Iout : Inport  Port=3
  Temp (Ra) : Inport  Port=4  Unit=degC
  Battery Core (w/ Q) : Subsystem
  Bus : Lib_PF_BusLoadDC_TMATS/LoadBus DC  P_M=0  BlkNm_M=double(gcb)
  Bus Creator : BusCreator  Inputs=7
  Gain : Gain  Gain=-1
  Mux : Mux  Inputs=2
  Product1 : Product
  Rankine to Celsius : $bdroot/Rankine to Celsius  SystemSampleTime=-1  VariantActivationTime=update diagram  Latency=0  AutoFrameSizeCalculation=off
  "TempConv " : Subsystem  Commented=on
      mask DialogControl DescTextVar Prompt: Temperature Unit Converter
  Terminator3 : Terminator
  it_Dot = f(i) : Subsystem
  Vout : Outport  VectorParamsAs1DForOutWhenUnconnected=off
  P_err : Outport  Port=2  VectorParamsAs1DForOutWhenUnconnected=off
  Outputs : Outport  Port=3  VectorParamsAs1DForOutWhenUnconnected=off
  it_Dot : Outport  Port=4  VectorParamsAs1DForOutWhenUnconnected=off
  Heat : Outport  Port=5  VectorParamsAs1DForOutWhenUnconnected=off
  wires:
  Rankine to Celsius/1 -> Battery Core (w/ Q)/3(Tavg)
  Battery Core (w/ Q)/3(it) -> Bus Creator/6  "it"
  Battery Core (w/ Q)/2(SOC) -> Bus Creator/4  "SOC"
  it_base/1 -> Battery Core (w/ Q)/1(it_base)
  Battery Core (w/ Q)/1(Vout) -> Bus Creator/1, Product1/1, Bus/1  "Vout"
  Product1/1 -> Bus Creator/3  "Pout"
  [Iout] -> Mux/1
  Gain/1 -> Mux/2
  Bus/2 -> P_err/1
  Bus/3 -> Terminator3/1
  Iout/1 -> it_Dot = f(i)/1(i), [Iout]
  Bus/1 -> Vout/1
  Mux/1 -> Bus/2
  it_Dot = f(i)/1(it_Dot) -> Bus Creator/5, it_Dot/1  "it_Dot"
  IgIn/1 -> Battery Core (w/ Q)/2(IgIn), Gain/1, Product1/2, Bus Creator/2  "Iout"
  Bus Creator/1 -> Outputs/1
  Battery Core (w/ Q)/4(Heat_Generated) -> Heat/1, Bus Creator/7  "Heat_Generated"
  Temp (Ra)/1 -> Rankine to Celsius/1

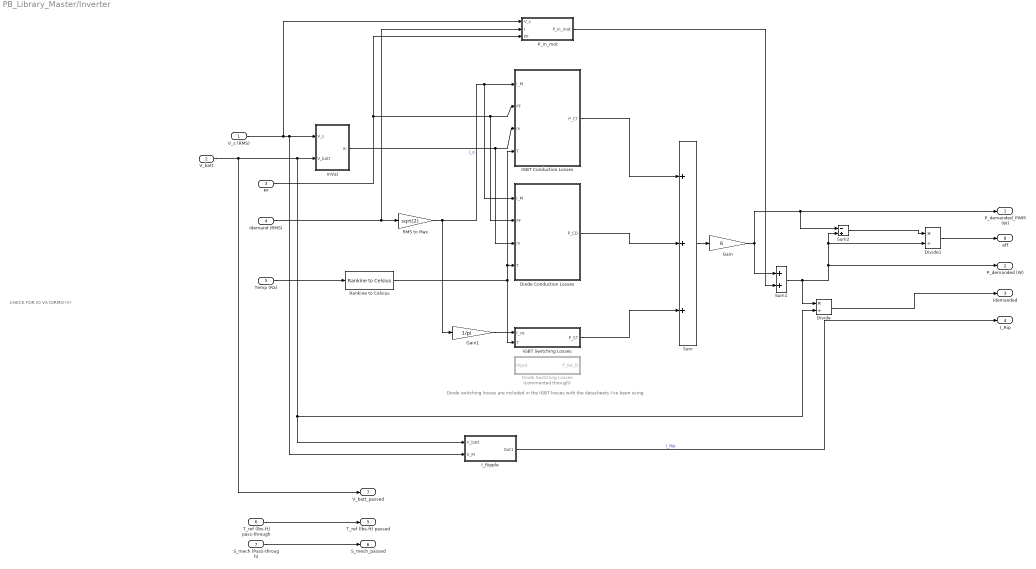
== system PB_Library_Master/Inverter ==
  note: Diode switching losses are included in the IGBT losses with the datasheets I've been using
  note: CHECK FOR IO VS IORMS!!!!!
  "V_s (RMS) " : Inport
  V_batt : Inport  Port=2
  PF : Inport  Port=3
  Idemand (RMS) : Inport  Port=4
  Temp (Ra) : Inport  Port=5
  T_ref (lbs-ft) pass-through : Inport  Port=6
  S_mech (Pass-through) : Inport  Port=7
  Diode Conduction Losses : Subsystem
  Diode Switching Losses : Subsystem  Commented=through
  Divide : Product  Inputs=*/
  Divide1 : Product  Inputs=*/
  Gain : Gain  Gain=6
  Gain1 : Gain  Gain=1/pi
  IGBT Conduction Losses : Subsystem
  IGBT Switching Losses : Subsystem
  I_Ripple : Subsystem
  P_in_mot : Subsystem
  RMS to Max : Gain  Gain=sqrt(2)
  Rankine to Celsius : $bdroot/Rankine to Celsius  SystemSampleTime=-1  VariantActivationTime=update diagram  Latency=0  AutoFrameSizeCalculation=off
  Sum : Sum  Inputs=+++
  Sum1 : Sum
  Sum2 : Sum  Inputs=-+
  mVal : Subsystem
  P_demanded_PWM (W) : Outport  VectorParamsAs1DForOutWhenUnconnected=off
  P_demanded (W) : Outport  Port=2  VectorParamsAs1DForOutWhenUnconnected=off
  Idemanded : Outport  Port=3  VectorParamsAs1DForOutWhenUnconnected=off
  I_Rip : Outport  Port=4  VectorParamsAs1DForOutWhenUnconnected=off
  T_ref (lbs-ft) passed : Outport  Port=5  VectorParamsAs1DForOutWhenUnconnected=off
  S_mech_passed : Outport  Port=6  VectorParamsAs1DForOutWhenUnconnected=off
  V_batt_passed : Outport  Port=7  VectorParamsAs1DForOutWhenUnconnected=off
  eff : Outport  Port=8  VectorParamsAs1DForOutWhenUnconnected=off
  wires:
  Idemand (RMS)/1 -> P_in_mot/2(I), RMS to Max/1
  RMS to Max/1 -> Gain1/1, Diode Conduction Losses/1(I_M), IGBT Conduction Losses/1(I_M)  "I_o"
  V_batt/1 -> V_batt_passed/1, mVal/2(V_batt), I_Ripple/1(V_batt), Divide/2
  IGBT Conduction Losses/1(P_CT) -> Sum/1
  Sum/1 -> Gain/1
  Gain/1 -> Sum2/1, P_demanded_PWM (W)/1, Sum1/1
  PF/1 -> P_in_mot/3(PF), Diode Conduction Losses/2(PF), IGBT Conduction Losses/2(PF)
  mVal/1(m) -> Diode Conduction Losses/3(m), IGBT Conduction Losses/3(m)
  "V_s (RMS) "/1 -> P_in_mot/1(V_s), I_Ripple/2("V_M "), mVal/1(V_s)
  P_in_mot/1(P_in_mot) -> Sum1/2
  Divide/1 -> Idemanded/1
  Gain1/1 -> IGBT Switching Losses/1(I_ce)
  IGBT Switching Losses/1(P_ST) -> Sum/3
  Diode Conduction Losses/1(P_CD) -> Sum/2
  Temp (Ra)/1 -> Rankine to Celsius/1
  I_Ripple/1(Out1) -> I_Rip/1  "I_Rip"
  T_ref (lbs-ft) pass-through/1 -> T_ref (lbs-ft) passed/1
  S_mech (Pass-through)/1 -> S_mech_passed/1
  Sum1/1 -> Divide/1, Sum2/2, Divide1/2, P_demanded (W)/1
  Sum2/1 -> Divide1/1
  Divide1/1 -> eff/1
  Rankine to Celsius/1 -> IGBT Switching Losses/2(T), Diode Conduction Losses/4(T), IGBT Conduction Losses/4(T)
